simulink model "FM"  (R2016a)
settings: Solver=VariableStepAuto  StartTime=0.0  StopTime=10.0  RelTol=1e-3
undefined symbols (not defined in the file): DiscIntNeverNeededParam
libraries: dspsrcs4 x1
settings Model: Creator=Student  LastModifiedBy=Student

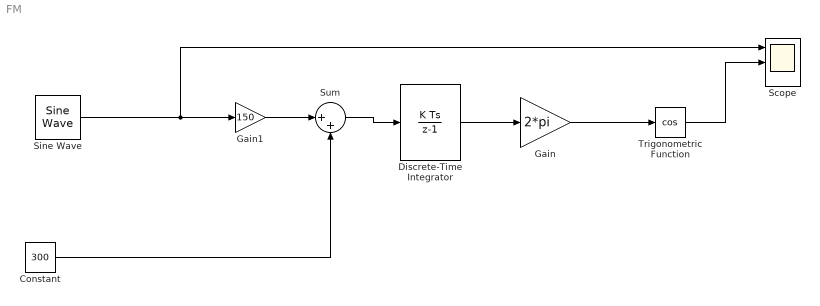
== system FM ==
  Constant : Constant  Value=300
  Discrete-Time Integrator : DiscreteIntegrator  InitialConditionSetting=State (most efficient)  SampleTime=1/98000  ICPrevOutput=DiscIntNeverNeededParam  ICPrevScaledInput=DiscIntNeverNeededParam
  Gain : Gain  Gain=2*pi
  Gain1 : Gain  Gain=150
  Scope : Scope  NumInputPorts=3
  Sine Wave : dspsrcs4/Sine Wave  Amplitude=1  Frequency=10  Phase=90  SampleMode=Discrete  OutComplex=Real  CompMethod=Trigonometric fcn  TableSize=Speed  SampleTime=1/98000  SamplesPerFrame=1  ResetState=Restart at time zero  OutputFrames=off  dataType=double  wordLen=16  udDataType=sfix(16)  fracBitsMode=Best precision  numFracBits=15  OutDataTypeStr=double  LastOutDataTypeStr=double
  Sum : Sum  Inputs=|++
  Trigonometric Function : Trigonometry  Operator=cos
  wires:
  Gain1/1 -> Sum/1
  Discrete-Time Integrator/1 -> Gain/1
  Gain/1 -> Trigonometric Function/1
  Sum/1 -> Discrete-Time Integrator/1
  Constant/1 -> Sum/2
  Sine Wave/1 -> Scope/1, Gain1/1
  Trigonometric Function/1 -> Scope/2
